simulink model "velo_pi"  (R2021b)
settings: Solver=ode4  StartTime=0.0  StopTime=20  RelTol=1e-3  EnableMultiTasking=on
undefined symbols (not defined in the file or in its folder): ts
libraries: arduino_io_lib x5
settings Model: Creator=hirata  LastModifiedBy=is221042
settings SolverCC: AlgebraicLoopSolver=TrustRegion
settings DataIOCC: LimitDataPoints=on  SaveFormat=Array  SignalLoggingSaveFormat=ModelDataLogs  ReturnWorkspaceOutputs=off
settings OptimizationCC: ExpressionDepthLimit=2147483647  LifeSpan=inf
settings DebuggingCC: UnderspecifiedInitializationDetection=Classic  MergeDetectMultiDrivingBlocksExec=none  SolverPrmCheckMsg=warning  FcnCallInpInsideContextMsg=warning  StateNameClashWarn=warning  SFUnexpectedBacktrackingDiag=warning  SFNoUnconditionalDefaultTransitionDiag=warning  SFMachineParentedDataDiag=warning  ArithmeticOperatorsInVariantConditions=warning
settings HardwareCC: ProdBitPerPointer=32  ProdBitPerSizeT=32  ProdBitPerPtrDiffT=32  ProdLargestAtomicFloat=None  ProdIntDivRoundTo=Undefined  ProdEndianess=Unspecified  ProdWordSize=32  ProdHWDeviceType=32-bit Generic
settings ModelReferenceCC: PropagateSignalLabelsOutOfModel=off
settings SFSimCC: SimUseLocalCustomCode=off  CustomCodeUndefinedFunction=UseInterfaceOnly
settings RTWCC: RTWUseLocalCustomCode=off
settings CodeAppCC: StateflowObjectComments=on
settings GRTTargetCC: TargetLangStandard=C89/C90 (ANSI)
settings ConfigComp: CovMetricSettings=dw  CovSaveCumulativeToWorkspaceVar=on  CovSaveSingleToWorkspaceVar=on  CovExternalEMLEnable=off

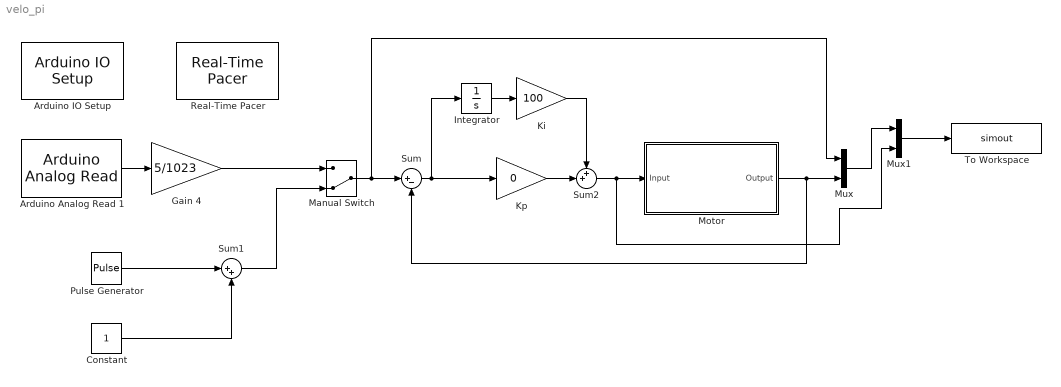
== system velo_pi ==
  Arduino Analog Read 1 : arduino_io_lib/Arduino Analog Read  arduinoVar=Temporary arduino variable: Arduino1  arduinoPin=1  T=ts
  Arduino IO Setup : arduino_io_lib/Arduino IO Setup  Priority=3  arduinoVar=Temporary arduino variable: Arduino1  workspaceVarName=a  comPort=/dev/ttyACM0
  Constant : Constant
  Gain 4 : Gain  Gain=5/1023
  Integrator : Integrator
  Ki : Gain  Gain=100
  Kp : Gain  Gain=0
  Manual Switch : ManualSwitch  CurrentSetting=0
  Motor : Subsystem
  Mux : Mux  Inputs=2
  Mux1 : Mux  Inputs=2
  Pulse Generator : DiscretePulseGenerator  Amplitude=0.5  Period=10/ts  PulseWidth=5/ts  SampleTime=ts
  Real-Time Pacer : arduino_io_lib/Real-Time Pacer  simTimePerRealTime=1
  Sum : Sum  Inputs=|+-
  Sum1 : Sum  Inputs=|++
  Sum2 : Sum  Inputs=++|
  To Workspace : ToWorkspace  VariableName=simout  SaveFormat=Timeseries  SampleTime=-1
  wires:
  Motor/1(Output) -> Mux/2, Sum/2
  Arduino Analog Read 1/1 -> Gain 4/1
  Sum2/1 -> Motor/1(Input), Mux1/2
  Sum/1 -> Kp/1, Integrator/1
  Manual Switch/1 -> Sum/1, Mux/1
  Gain 4/1 -> Manual Switch/1
  Constant/1 -> Sum1/2
  Pulse Generator/1 -> Sum1/1
  Sum1/1 -> Manual Switch/2
  Integrator/1 -> Ki/1
  Ki/1 -> Sum2/1
  Kp/1 -> Sum2/2
  Mux/1 -> Mux1/1
  Mux1/1 -> To Workspace/1

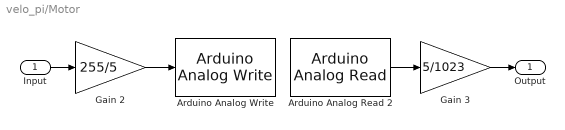
== system velo_pi/Motor ==
  Input : Inport
  Arduino Analog Read 2 : arduino_io_lib/Arduino Analog Read  arduinoVar=Temporary arduino variable: Arduino1  arduinoPin=0  T=ts
  Arduino Analog Write : arduino_io_lib/Arduino Analog Write  arduinoVar=Temporary arduino variable: Arduino1  arduinoPin=3  T=ts
  Gain 2 : Gain  Gain=255/5
  Gain 3 : Gain  Gain=5/1023
  Output : Outport
  wires:
  Arduino Analog Read 2/1 -> Gain 3/1
  Gain 2/1 -> Arduino Analog Write/1
  Input/1 -> Gain 2/1
  Gain 3/1 -> Output/1
